simulink model "MPC_VS_FOC"  (R2021a)
settings: Solver=VariableStepAuto  StartTime=0.0  StopTime=0.02  RelTol=1e-3
libraries: spsMosfetLib x12, spsCurrentMeasurementLib x3, spsPermanentMagnetSynchronousMachineLib x2, spsDCVoltageSourceLib x2, spsGroundLib x2, spsThreePhaseVIMeasurementLib x2, pid_lib x1, spsSVPWMGenerator2LevelLib x1, spsabctodq0Lib x1, spspowerguiLib x1
settings Model: Creator=Hassan Alam  LastModifiedBy=zero
settings SolverCC: ZeroCrossAlgorithm=Adaptive
settings DebuggingCC: MaskedZcDiagnostic=none  IgnoredZcDiagnostic=none  SFMachineParentedDataDiag=warning  ArithmeticOperatorsInVariantConditions=warning
settings SFSimCC: CustomCodeUndefinedFunction=UseInterfaceOnly

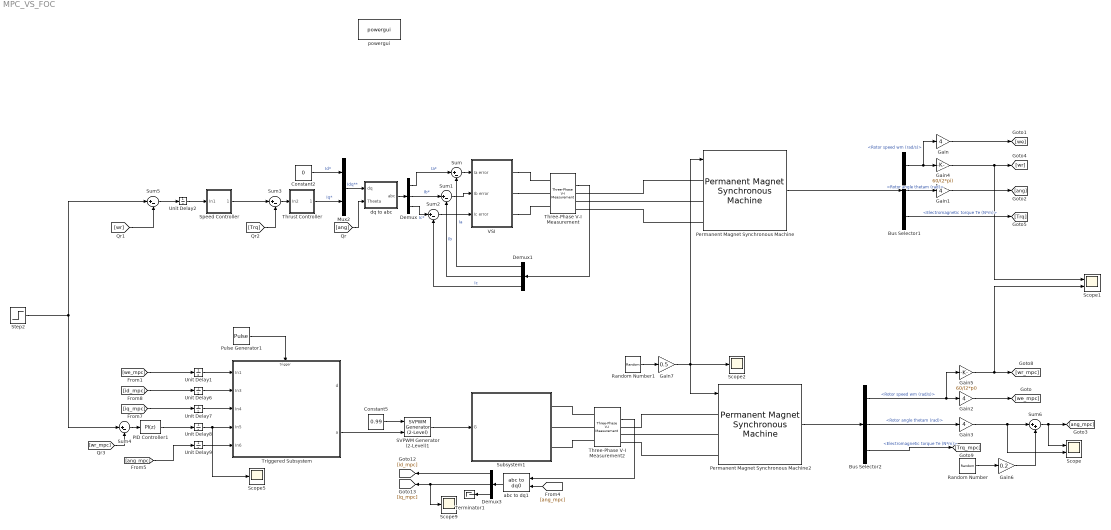
== system MPC_VS_FOC ==
  Bus Selector1 : BusSelector  OutputSignals=Rotor speed wm (rad/s),Rotor angle thetam (rad),Electromagnetic torque Te (N*m)
  Bus Selector2 : BusSelector  OutputSignals=Rotor speed wm (rad/s),Rotor angle thetam (rad),Electromagnetic torque Te (N*m)
  Constant2 : Constant  Value=0
  Constant5 : Constant  Value=0.99
  Demux : Demux  Outputs=3
  Demux1 : Demux  Outputs=3
  Demux3 : Demux  Outputs=3
  Gain{,1..3} (4 alike) : Gain  Gain=4  SaturateOnIntegerOverflow=on  OutDataTypeStr=Inherit: Same as input  ParamDataTypeStr=Inherit: Same as input
  Gain4 : Gain  Gain=60/(2*pi)  SaturateOnIntegerOverflow=on  OutDataTypeStr=Inherit: Same as input  ParamDataTypeStr=Inherit: Same as input
  Gain5 : Gain  Gain=60/(2*pi)  SaturateOnIntegerOverflow=on  OutDataTypeStr=Inherit: Same as input  ParamDataTypeStr=Inherit: Same as input
  Gain6 : Gain  Gain=0.2
  Gain7 : Gain  Gain=0.5
  Mux2 : Mux  Inputs=2
  PID Controller1 : pid_lib/PID Controller  Controller=PI  Form=Parallel  TimeDomain=Discrete-time  UseExternalTs=off  SampleTime=50e-6  IntegratorMethod=Forward Euler  FilterMethod=Forward Euler  ControllerParametersSource=internal  P=0.05  I=1  D=5  UseFilter=on  N=100  TunerSelectOption=Transfer Function Based (PID Tuner App)  InitialConditionSource=internal  InitialConditionForIntegrator=0  InitialConditionForFilter=0  DifferentiatorICPrevScaledInput=0  ExternalReset=none  TrackingMode=off  Kt=1  LimitOutput=off  SatLimitsSource=internal  UpperSaturationLimit=0.6  LowerSaturationLimit=-0.6  LinearizeAsGain=on  AntiWindupMode=clamping  Kb=1  RndMeth=Nearest  POutMin=[]  POutMax=[]  IOutMin=[]  IOutMax=[]  DOutMin=[]  DOutMax=[]  NOutMin=[]  NOutMax=[]  SumOutMin=[]  SumOutMax=[]  SaturationOutMin=[]  SaturationOutMax=[]  PParamMin=[]  PParamMax=[]  IParamMin=[]  IParamMax=[]  DParamMin=[]  DParamMax=[]  NParamMin=[]  NParamMax=[]  KbParamMin=[]  KbParamMax=[]  KtParamMin=[]  KtParamMax=[]  KbOutMin=[]  KbOutMax=[]  KtOutMin=[]  KtOutMax=[]  IntegratorOutMin=[]  IntegratorOutMax=[]  FilterOutMin=[]  FilterOutMax=[]  SumI1OutMin=[]  SumI1OutMax=[]  SumI2OutMin=[]  SumI2OutMax=[]  SumI3OutMin=[]  SumI3OutMax=[]  SumI4OutMin=[]  SumI4OutMax=[]  SumDOutMin=[]  SumDOutMax=[]  DifferentiatorOutMin=[]  DifferentiatorOutMax=[]  FilterDiffOutCoefMin=[]  FilterDiffOutCoefMax=[]  ReciprocalOutMin=[]  ReciprocalOutMax=[]  SumDenOutMin=[]  SumDenOutMax=[]  SumNumOutMin=[]  SumNumOutMax=[]  DivideOutMin=[]  DivideOutMax=[]  UdiffTsProdOutMin=[]  UdiffTsProdOutMax=[]  NTsProdOutMin=[]  NTsProdOutMax=[]  UintegralTsProdOutMin=[]  UintegralTsProdOutMax=[]  UngainTsProdOutMin=[]  UngainTsProdOutMax=[]  IntegratorContinuousStateAttributes=''  IntegratorStateMustResolveToSignalObject=off  IntegratorRTWStateStorageClass=Auto  FilterContinuousStateAttributes=''  FilterStateMustResolveToSignalObject=off  FilterRTWStateStorageClass=Auto  ParallelPVariant=InternalParameters  IdealPVariant=Disabled  IVariant=InternalParameters  DVariant=Disabled  IntegratorVariant=Discrete  SatVariant=Disabled  AWVariant=Passthrough  PCopyVariant=Disabled  TRVariant=Disabled  FdbkBlocksVariant=Forward  IdealPFdbkVariant=Disabled  SatFdbkVariant=Disabled  DerivativeFilterVariant=Disabled  NVariant=Disabled  NCopyVariant=Disabled_SignalSpec  FilterICVariant=Disabled  IntegratorICVariant=InternalICs  ExternalResetVariant=Disabled  TRSumVariant=Passthrough  SumFdbkVariant=Disabled  SumVariant=Sum_PI  TsampFilterVariant=InternalTs  TsampNgainVariant=Passthrough  TsampIntegralVariant=Passthrough  ExternalSaturationOutDataTypeStr=Inherit: Same as second input
  Permanent Magnet Synchronous Machine : spsPermanentMagnetSynchronousMachineLib/Permanent Magnet Synchronous Machine  NbPhases=3  FluxDistribution=Trapezoidal  RotorType=Round  MechanicalLoad=Torque Tm  PresetModel=No  ShowDetailedParameters=on  MeasurementBus=off  Resistance=0.375  Inductance=0.0002  dqInductances=[8.5e-3,8.5e-3]  La=0.0002  MachineConstant=Flux linkage established by magnets (V.s)  Flux=0.0066667  VoltageCst=5.5851  TorqueCst=0.053334  Flat=120  Mechanical=[2.66e-6 1.3e-6 4 0]  PolePairs=4  InitialConditions=[0,0, 0,0]  InitialConditions5ph=[0 0 0 0 0 0]  RefAngle=Aligned with phase A axis (original Park)  IterativeDiscreteModel=Trapezoidal non iterative  TsBlock=-1  TsPowergui=0
  Permanent Magnet Synchronous Machine2 : spsPermanentMagnetSynchronousMachineLib/Permanent Magnet Synchronous Machine  NbPhases=3  FluxDistribution=Trapezoidal  RotorType=Round  MechanicalLoad=Torque Tm  PresetModel=No  ShowDetailedParameters=on  MeasurementBus=off  Resistance=0.375  Inductance=0.0002  dqInductances=[8.5e-3,8.5e-3]  La=0.0002  MachineConstant=Flux linkage established by magnets (V.s)  Flux=0.0066667  VoltageCst=5.5851  TorqueCst=0.053334  Flat=120  Mechanical=[2.66e-6 1.3e-6 4 0]  PolePairs=4  InitialConditions=[0,0, 0,0]  InitialConditions5ph=[0 0 0 0 0 0]  RefAngle=90 degrees behind phase A axis (modified Park)  IterativeDiscreteModel=Trapezoidal non iterative  TsBlock=-1  TsPowergui=0
  Pulse Generator1 : DiscretePulseGenerator  PulseType=Time based  Period=50e-6  PulseWidth=5
  Random Number : RandomNumber  Mean=0.1  SampleTime=30e-6
  Random Number1 : RandomNumber  Mean=0.1  SampleTime=30e-6
  SVPWM Generator (2-Level)1 : spsSVPWMGenerator2LevelLib/SVPWM Generator (2-Level)  InputType=Magnitude-Angle (rad)  SwitchingPattern=Pattern #1  Fc=30000  ParUref=[0.8 -30 50]  Ts=0
      settings: SourceProductBaseCode=PS
  Scope : Scope  NumInputPorts=2
  Scope1 : Scope  NumInputPorts=2
  Scope2 : Scope
  Scope5 : Scope
  Scope9 : Scope
  Speed Controller : Subsystem
  Step2 : Step  Time=0.00  After=1600  SampleTime=0
  Subsystem1 : Subsystem
  Sum{,1..5} (6 alike) : Sum  Inputs=|+-
  Sum6 : Sum  Inputs=|++
  Terminator1 : Terminator
  Three-Phase V-I Measurement : spsThreePhaseVIMeasurementLib/Three-Phase V-I Measurement  VoltageMeasurement=phase-to-phase  SetLabelV=off  LabelV=Vabc  Vpu=off  VpuLL=off  CurrentMeasurement=yes  SetLabelI=off  LabelI=Iabc  Ipu=off  Pbase=100e6  Vbase=500e3  OutputType=Complex  PhasorSimulation=off  PSBequivalent=0
  Three-Phase V-I Measurement2 : spsThreePhaseVIMeasurementLib/Three-Phase V-I Measurement  VoltageMeasurement=phase-to-phase  SetLabelV=off  LabelV=Vabc  Vpu=off  VpuLL=off  CurrentMeasurement=yes  SetLabelI=off  LabelI=Iabc  Ipu=off  Pbase=100e6  Vbase=500e3  OutputType=Complex  PhasorSimulation=off  PSBequivalent=0
  Thrust Controller : Subsystem
  Triggered Subsystem : Subsystem  TreatAsAtomicUnit=on
  Unit Delay{1..2,6..9} (6 alike) : UnitDelay  SampleTime=-1  HasFrameUpgradeWarning=on
  VSI : Subsystem
  abc to dq1 : spsabctodq0Lib/abc to dq0  Alignment=90 degrees behind phase A axis
  dq to abc : Subsystem
  powergui : spspowerguiLib/powergui  Priority=1  SimulationMode=Discrete  SampleTime=3e-7  frequency=60  Iterations=50  frequencyindice=0  Pbase=100e6  ErrMax=1e-4  UnitsV=kV  UnitsW=MW  buscounter=0  FunctionMessages=off  echomessages=off  EnableUseOfTLC=off  CurrentSourceSwitches=off  DisableSnubberDevices=off  DisableRonSwitches=off  DisableVfSwitches=off  DisplayEquations=off  AutomaticDiscreteSolvers=off  SolverType=Tustin/Backward Euler (TBE)  Interpol=off  ExternalGateDelay=off  methode=off  Ts=100  x0status=blocks  SPID=on  SwTol=0  HookPort=off  NonlinearTolerance=1e-4  nMaxIteration=100  ContinueOnMaxIteration=off  RestoreLinks=warning  ResistiveCurrentMeasurement=off  Frange=[0:2:500]  Ylog=off  Xlog=on  ShowGrid=off  save=off  variable=ZData  structure=0  ZoomFFT=off  StartTime=0.0  cycles=1  DisplayStyle=1  fundamental=60  FreqAxis=off  MaxFrequency=1000  frequencyindicesteady=1  RmsSteady=1  display=off
  wires:
  Sum2/1 -> VSI/3(Ic error)
  Sum1/1 -> VSI/2(Ib error)
  Sum/1 -> VSI/1(Ia error)
  dq to abc/1(abc) -> Demux/1
  Demux/2 -> Sum1/1  "Ib*"
  Demux/1 -> Sum/1  "Ia*"
  Demux/3 -> Sum2/1  "Ic*"
  Thrust Controller/1(Out2) -> Mux2/2  "Iq*"
  Constant2/1 -> Mux2/1  "Id*"
  Mux2/1 -> dq to abc/1(dq)  "Idq**"
  Demux1/1 -> Sum/2  "Ia"
  Demux1/2 -> Sum1/2  "Ib"
  Demux1/3 -> Sum2/2  "Ic"
  Speed Controller/1(Out1) -> Sum3/1
  [ang] -> dq to abc/2(Theeta)
  Sum5/1 -> Unit Delay2/1
  Sum3/1 -> Thrust Controller/1(In2)
  Step2/1 -> Sum4/1, Sum5/1
  Bus Selector1/2 -> Gain1/1  "<Rotor angle thetam (rad)>"
  Permanent Magnet Synchronous Machine/1 -> Bus Selector1/1
  Bus Selector1/1 -> Gain/1, Gain4/1  "<Rotor speed wm (rad/s)>"
  Gain4/1 -> Scope1/1, [wr]
  Gain1/1 -> [ang]
  Gain/1 -> [we]
  Bus Selector1/3 -> [Trq]  "<Electromagnetic torque Te (N*m)>"
  Random Number1/1 -> Gain7/1
  Three-Phase V-I Measurement/2 -> Demux1/1
  [wr] -> Sum5/2
  [Trq] -> Sum3/2
  Bus Selector2/2 -> Gain3/1  "<Rotor angle thetam (rad)>"
  Bus Selector2/1 -> Gain5/1, Gain2/1  "<Rotor speed wm (rad/s)>"
  Gain5/1 -> Scope1/2, [wr_mpc]
  Bus Selector2/3 -> [Trq_mpc]  "<Electromagnetic torque Te (N*m)>"
  Gain2/1 -> [we_mpc]
  Unit Delay7/1 -> Triggered Subsystem/3(In4)
  Triggered Subsystem/2(a) -> SVPWM Generator (2-Level)1/2
  [we_mpc] -> Unit Delay1/1
  Pulse Generator1/1 -> Triggered Subsystem/Trigger
  Constant5/1 -> SVPWM Generator (2-Level)1/1
  [ang_mpc] -> Unit Delay9/1
  [iq_mpc] -> Unit Delay7/1
  Sum4/1 -> PID Controller1/1
  Demux3/2 -> Scope9/1, [iq_mpc]
  SVPWM Generator (2-Level)1/1 -> Subsystem1/1(G)
  PID Controller1/1 -> Unit Delay8/1
  Demux3/1 -> [id_mpc]
  Demux3/3 -> Terminator1/1
  Unit Delay8/1 -> Scope5/1, Triggered Subsystem/4(In5)
  Three-Phase V-I Measurement2/2 -> abc to dq1/1
  Unit Delay1/1 -> Triggered Subsystem/1(In1)
  [id_mpc] -> Unit Delay6/1
  [ang_mpc] -> abc to dq1/2
  [wr_mpc] -> Sum4/2
  Unit Delay6/1 -> Triggered Subsystem/2(In3)
  Unit Delay9/1 -> Triggered Subsystem/5(In6)
  abc to dq1/1 -> Demux3/1
  Permanent Magnet Synchronous Machine2/1 -> Bus Selector2/1
  Unit Delay2/1 -> Speed Controller/1(In1)
  Gain3/1 -> Scope/2, Sum6/1
  Random Number/1 -> Gain6/1
  Sum6/1 -> Scope/1, [ang_mpc]
  Gain6/1 -> Sum6/2
  Gain7/1 -> Permanent Magnet Synchronous Machine/1, Scope2/1, Permanent Magnet Synchronous Machine2/1
  connections:
  Permanent Magnet Synchronous Machine/LConn3 -- Three-Phase V-I Measurement/RConn3
  Permanent Magnet Synchronous Machine/LConn1 -- Three-Phase V-I Measurement/RConn1
  Permanent Magnet Synchronous Machine/LConn2 -- Three-Phase V-I Measurement/RConn2
  VSI/RConn1 -- Three-Phase V-I Measurement/LConn1
  VSI/RConn2 -- Three-Phase V-I Measurement/LConn2
  VSI/RConn3 -- Three-Phase V-I Measurement/LConn3
  Three-Phase V-I Measurement2/LConn2 -- Subsystem1/RConn2
  Three-Phase V-I Measurement2/LConn1 -- Subsystem1/RConn1
  Three-Phase V-I Measurement2/LConn3 -- Subsystem1/RConn3
  Permanent Magnet Synchronous Machine2/LConn1 -- Three-Phase V-I Measurement2/RConn1
  Permanent Magnet Synchronous Machine2/LConn3 -- Three-Phase V-I Measurement2/RConn3
  Permanent Magnet Synchronous Machine2/LConn2 -- Three-Phase V-I Measurement2/RConn2

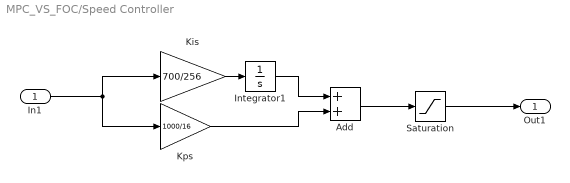
== system MPC_VS_FOC/Speed Controller ==
  In1 : Inport
  Add : Sum
  Integrator1 : Integrator
  Kis : Gain  Gain=700/256
  Kps : Gain  Gain=1000/16
  Saturation : Saturate  UpperLimit=50  LowerLimit=-50
  Out1 : Outport
  wires:
  Saturation/1 -> Out1/1
  Kps/1 -> Add/2
  In1/1 -> Kis/1, Kps/1
  Kis/1 -> Integrator1/1
  Add/1 -> Saturation/1
  Integrator1/1 -> Add/1

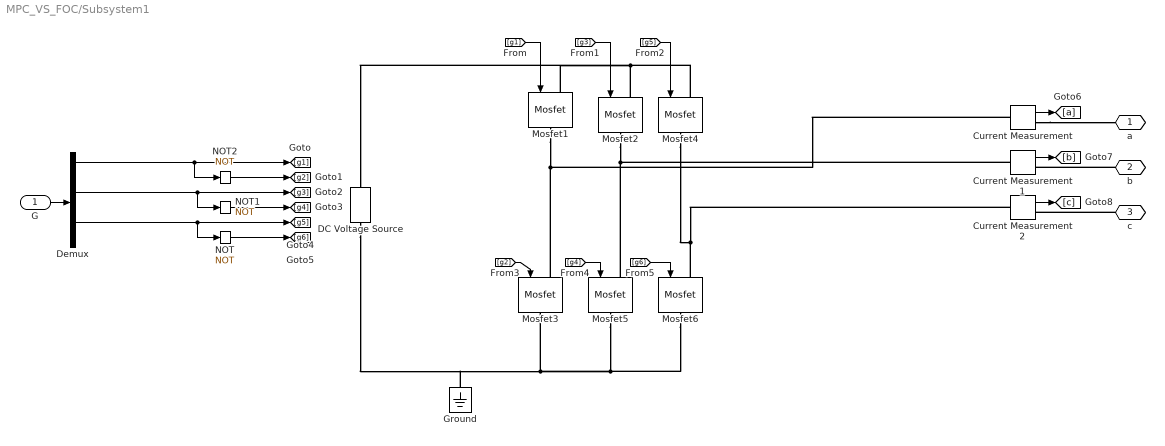
== system MPC_VS_FOC/Subsystem1 ==
  G : Inport
  Current Measurement : spsCurrentMeasurementLib/Current Measurement  PhasorSimulation=off  OutputType=Complex  PSBequivalent=0
  Current Measurement1 : spsCurrentMeasurementLib/Current Measurement  PhasorSimulation=off  OutputType=Complex  PSBequivalent=0
  Current Measurement2 : spsCurrentMeasurementLib/Current Measurement  PhasorSimulation=off  OutputType=Complex  PSBequivalent=0
  DC Voltage Source : spsDCVoltageSourceLib/DC Voltage Source  Amplitude=12  Measurements=None
  Demux : Demux  Outputs=6
  Ground : spsGroundLib/Ground  LConnTagsString=a
  Mosfet{1..6} (6 alike) : spsMosfetLib/Mosfet  Ron=0.001  Lon=0  Rd=0.001  Vfd=0  IC=0  Rs=1e5  Cs=inf  Measurements=off
  NOT : Logic  Operator=NOT  IconShape=distinctive  AllPortsSameDT=off  OutDataTypeStr=boolean
  NOT1 : Logic  Operator=NOT  IconShape=distinctive  AllPortsSameDT=off  OutDataTypeStr=boolean
  NOT2 : Logic  Operator=NOT  IconShape=distinctive  AllPortsSameDT=off  OutDataTypeStr=boolean
  a : PMIOPort  Side=Right
  b : PMIOPort  Port=2  Side=Right
  c : PMIOPort  Port=3  Side=Right
  wires:
  [g3] -> Mosfet2/1
  [g4] -> Mosfet5/1
  [g2] -> Mosfet3/1
  [g6] -> Mosfet6/1
  [g5] -> Mosfet4/1
  [g1] -> Mosfet1/1
  Demux/5 -> NOT/1, [g5]
  G/1 -> Demux/1
  Demux/3 -> NOT1/1, [g3]
  Demux/1 -> NOT2/1, [g1]
  NOT/1 -> [g6]
  NOT1/1 -> [g4]
  NOT2/1 -> [g2]
  Current Measurement/1 -> [a]
  Current Measurement1/1 -> [b]
  Current Measurement2/1 -> [c]
  connections:
  Current Measurement/LConn1 -- Mosfet1/RConn1 -- Mosfet3/LConn1
  Current Measurement1/LConn1 -- Mosfet5/LConn1 -- Mosfet2/RConn1
  Current Measurement2/LConn1 -- Mosfet6/LConn1 -- Mosfet4/RConn1
  DC Voltage Source/LConn1 -- Ground/LConn1 -- Mosfet3/RConn1 -- Mosfet6/RConn1 -- Mosfet5/RConn1
  Mosfet1/LConn1 -- DC Voltage Source/RConn1 -- Mosfet4/LConn1 -- Mosfet2/LConn1
  Current Measurement/RConn1 -- a/RConn1
  b/RConn1 -- Current Measurement1/RConn1
  c/RConn1 -- Current Measurement2/RConn1

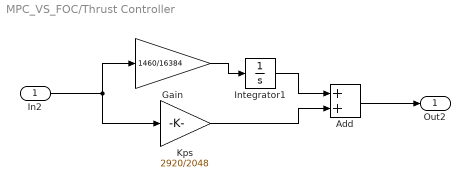
== system MPC_VS_FOC/Thrust Controller ==
  In2 : Inport
  Add : Sum
  Gain : Gain  Gain=1460/16384
  Integrator1 : Integrator
  Kps : Gain  Gain=2920/2048
  Out2 : Outport
  wires:
  In2/1 -> Gain/1, Kps/1
  Integrator1/1 -> Add/1
  Add/1 -> Out2/1
  Kps/1 -> Add/2
  Gain/1 -> Integrator1/1

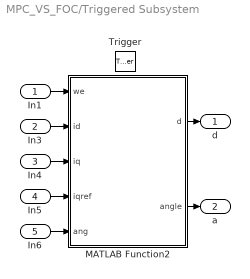
== system MPC_VS_FOC/Triggered Subsystem ==
  In1 : Inport
  In3 : Inport  Port=2
  In4 : Inport  Port=3
  In5 : Inport  Port=4
  In6 : Inport  Port=5
  Trigger : TriggerPort  VariantControl=Variant
  MATLAB Function2 : MATLAB Function  TreatAsAtomicUnit=on
  d : Outport  VectorParamsAs1DForOutWhenUnconnected=off
  a : Outport  Port=2  VectorParamsAs1DForOutWhenUnconnected=off
  wires:
  In1/1 -> MATLAB Function2/1(we)
  In3/1 -> MATLAB Function2/2(id)
  In4/1 -> MATLAB Function2/3(iq)
  In5/1 -> MATLAB Function2/4(iqref)
  In6/1 -> MATLAB Function2/5(ang)
  MATLAB Function2/1(d) -> d/1
  MATLAB Function2/2(angle) -> a/1

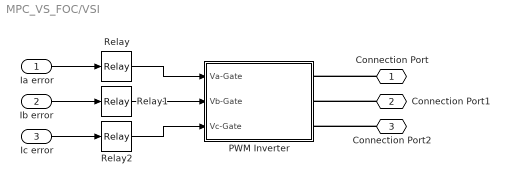
== system MPC_VS_FOC/VSI ==
  Ia error : Inport
  Ib error : Inport  Port=2
  Ic error : Inport  Port=3
  PWM Inverter : Subsystem
  Relay : Relay  OnSwitchValue=0.1  OffSwitchValue=-0.1
  Relay1 : Relay  OnSwitchValue=0.1  OffSwitchValue=-0.1
  Relay2 : Relay  OnSwitchValue=0.1  OffSwitchValue=-0.1
  Connection Port : PMIOPort  Side=Right
  Connection Port1 : PMIOPort  Port=2  Side=Right
  Connection Port2 : PMIOPort  Port=3  Side=Right
  wires:
  Ia error/1 -> Relay/1
  Ib error/1 -> Relay1/1
  Ic error/1 -> Relay2/1
  Relay1/1 -> PWM Inverter/2(Vb-Gate)
  Relay/1 -> PWM Inverter/1(Va-Gate)
  Relay2/1 -> PWM Inverter/3(Vc-Gate)
  connections:
  Connection Port/RConn1 -- PWM Inverter/RConn1
  Connection Port1/RConn1 -- PWM Inverter/RConn2
  Connection Port2/RConn1 -- PWM Inverter/RConn3

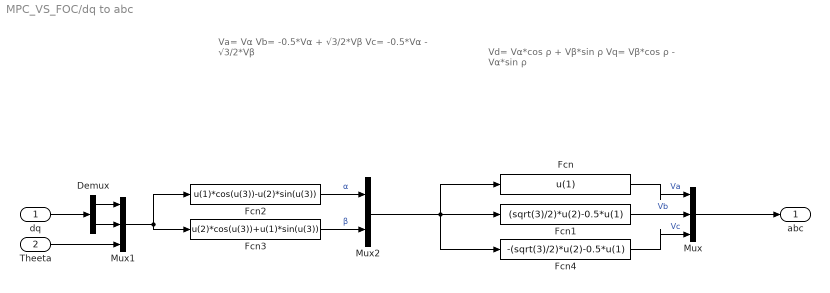
== system MPC_VS_FOC/dq to abc ==
  note: Va= Vα
      | Vb= -0.5*Vα + √3/2*Vβ
      | Vc= -0.5*Vα - √3/2*Vβ
  note: Vd= Vα*cos ρ + Vβ*sin ρ
      |
      | Vq= Vβ*cos ρ - Vα*sin ρ
  dq : Inport
  Theeta : Inport  Port=2
  Demux : Demux  Outputs=2
  Fcn : Fcn  Expr=u(1)
  Fcn1 : Fcn  Expr=(sqrt(3)/2)*u(2)-0.5*u(1)
  Fcn2 : Fcn  Expr=u(1)*cos(u(3))-u(2)*sin(u(3))
  Fcn3 : Fcn  Expr=u(2)*cos(u(3))+u(1)*sin(u(3))
  Fcn4 : Fcn  Expr=-(sqrt(3)/2)*u(2)-0.5*u(1)
  Mux : Mux  Inputs=3
  Mux1 : Mux  Inputs=3
  Mux2 : Mux  Inputs=2
  abc : Outport
  wires:
  Fcn/1 -> Mux/1  "Va"
  Fcn1/1 -> Mux/2  "Vb"
  Mux2/1 -> Fcn/1, Fcn4/1, Fcn1/1
  Fcn2/1 -> Mux2/1  "α"
  Fcn3/1 -> Mux2/2  "β"
  Theeta/1 -> Mux1/3
  Fcn4/1 -> Mux/3  "Vc"
  dq/1 -> Demux/1
  Mux1/1 -> Fcn3/1, Fcn2/1
  Demux/1 -> Mux1/1
  Demux/2 -> Mux1/2
  Mux/1 -> abc/1

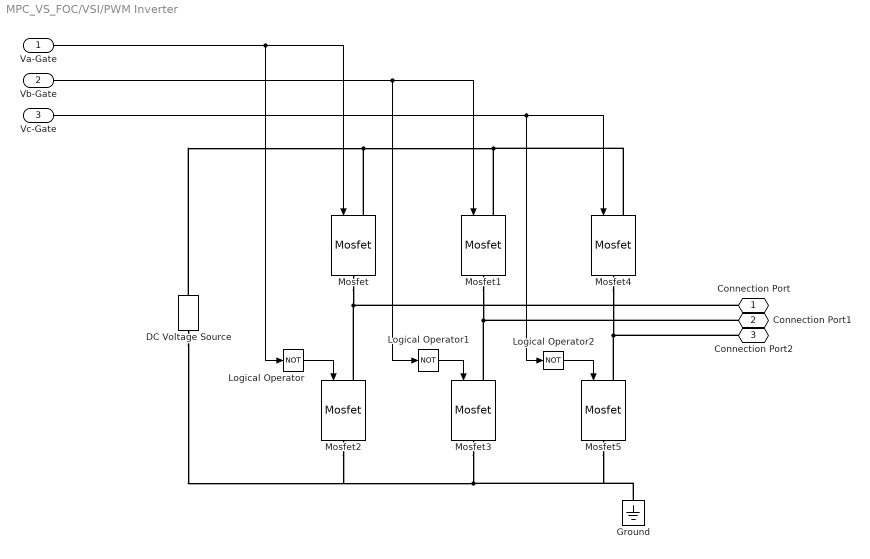
== system MPC_VS_FOC/VSI/PWM Inverter ==
  Va-Gate : Inport
  Vb-Gate : Inport  Port=2
  Vc-Gate : Inport  Port=3
  DC Voltage Source : spsDCVoltageSourceLib/DC Voltage Source  Amplitude=12  Measurements=None
  Ground : spsGroundLib/Ground  LConnTagsString=a
  Logical Operator : Logic  Operator=NOT  AllPortsSameDT=off  OutDataTypeStr=boolean
  Logical Operator1 : Logic  Operator=NOT  AllPortsSameDT=off  OutDataTypeStr=boolean
  Logical Operator2 : Logic  Operator=NOT  AllPortsSameDT=off  OutDataTypeStr=boolean
  Mosfet{,1..5} (6 alike) : spsMosfetLib/Mosfet  Ron=0.001  Lon=0  Rd=0.001  Vfd=0  IC=0  Rs=1e5  Cs=inf  Measurements=off
  Connection Port : PMIOPort  Side=Right
  Connection Port1 : PMIOPort  Port=2  Side=Right
  Connection Port2 : PMIOPort  Port=3  Side=Right
  wires:
  Logical Operator1/1 -> Mosfet3/1
  Logical Operator/1 -> Mosfet2/1
  Logical Operator2/1 -> Mosfet5/1
  Vc-Gate/1 -> Mosfet4/1, Logical Operator2/1
  Vb-Gate/1 -> Mosfet1/1, Logical Operator1/1
  Va-Gate/1 -> Logical Operator/1, Mosfet/1
  connections:
  Mosfet/LConn1 -- DC Voltage Source/RConn1 -- Mosfet4/LConn1 -- Mosfet1/LConn1
  Connection Port1/RConn1 -- Mosfet3/LConn1 -- Mosfet1/RConn1
  Mosfet/RConn1 -- Mosfet2/LConn1 -- Connection Port/RConn1
  Connection Port2/RConn1 -- Mosfet5/LConn1 -- Mosfet4/RConn1
  Mosfet2/RConn1 -- DC Voltage Source/LConn1 -- Mosfet3/RConn1 -- Mosfet5/RConn1 -- Ground/LConn1

== matlab function MPC_VS_FOC/Triggered Subsystem/MATLAB Function2 ==
  data: we input; id input; iq input; iqref input; ang input; d output; angle output
function [d,angle]  = MPC(we,id,iq,iqref,ang)

persistent oldState;

if isempty(oldState)
    oldState = 1;
end

Ts = 50e-6;
Vdc = 12;
L = 0.0002;
R = 0.375;
psiPM = 0.00666;

p = 0.7;
q = 0.4;
r = 0.6;
s = 0.8;

states =[1     0     0;
         1     1     0;
         0     1     0;
         0     1     1;
         0     0     1;
         1     0     1]*0.99;
%          p 0     0 p     0 p;
%          p 0     p 0     0 p;
%          0 p     p 0     0 p;
%          0 p     p 0     p 0;
%          0 p     0 p     p 0;
%          p 0     0 p     p 0;
%          q 0     0 q     0 q;
%          q 0     q 0     0 q;
%          0 q     q 0     0 q;
%          0 q     q 0     q 0;
%          0 q     0 q     q 0;
%          q 0     0 q     q 0;
%          r 0     0 r     0 r;
%          r 0     r 0     0 r;
%          0 r     r 0     0 r;
%          0 r     r 0     r 0;
%          0 r     0 r     r 0;
%          r 0     0 r     r 0;
%          s 0     0 s     0 s;
%          s 0     s 0     0 s;
%          0 s     s 0     0 s;
%          0 s     s 0     s 0;
%          0 s     0 s     s 0;
%          s 0     0 s     s 0;];

y = states(1,:)';
cost = [];

% id = (2/3)*[sin(ang) sin(ang - (2*pi/3)) sin(ang + (2*pi/3))]*[Iab(1) Iab(2) -(Iab(1)+Iab(2))]';
% iq = (2/3)*[cos(ang) cos(ang - (2*pi/3)) cos(ang + (2*pi/3))]*[Iab(1) Iab(2) -(Iab(1)+Iab(2))]';

for i=1:length(states)
    vsd = (2*Vdc/3)*[sin(ang) sin(ang - (2*pi/3)) sin(ang + (2*pi/3))]*states(i,[1,2,3])';
    vsq = (2*Vdc/3)*[cos(ang) cos(ang - (2*pi/3)) cos(ang + (2*pi/3))]*states(i,[1,2,3])';

    id_p = id;
    iq_p = iq;

    for x = 1:8
        id_p = ((1-(R*Ts/L))*id_p)+(Ts*we*iq_p)+(vsd*Ts/L);
        iq_p = ((1-(R*Ts/L))*iq_p)-(Ts*we*id_p)-(psiPM*we*Ts)+(vsq*Ts/L);
    end

    cost = [cost (id_p)^2 + (iqref - iq_p)^2];
end

a = find(cost == min(cost));
a = a(1);

d = 0.95;
angle = (a-1)*pi/3;
